simulink model "lab_hall"  (R2024b)
settings: Solver=FixedStepAuto  StartTime=0.0  StopTime=inf  FixedStep=0.001  RelTol=1e-3  EnableMultiTasking=on
libraries: stm32f4xxblockslib x2, simulink x1
settings Model: STM32="{\"AnalogInput\":[{\"ID\":\"lab_1:1\"},{\"ID\":\"lab_hall:1\"}],\"DigitalPortRead\":[{\"ID\":\"lab_1:126\"},{\"ID\":\"lab_hall:126\"}]}"  Creator=A1nz_01  LastModifiedBy=A1nz_01
settings OptimizationCC: EnhancedBackFolding=on  PassReuseOutputArgsAs=Individual arguments  ZeroExternalMemoryAtStartup=off  ZeroInternalMemoryAtStartup=off  MaxStackSize=64  OptimizeBlockOrder=speed  DifferentSizesBufferReuse=on  OptimizationCustomize=off  EfficientTunableParamExpr=on
settings DebuggingCC: ParameterTunabilityLossMsg=error
settings HardwareCC: ProdBitPerPointer=32  ProdBitPerSizeT=32  ProdBitPerPtrDiffT=32  ProdLargestAtomicInteger=Long  ProdLargestAtomicFloat=Double  ProdWordSize=32  ProdLongLongMode=on  ProdHWDeviceType=ARM Compatible->ARM Cortex-M
settings SFSimCC: MATLABDynamicMemAlloc=off
settings RTWCC: Description=Embedded Coder  SystemTargetFile=ert.tlc  HardwareBoard=STM32G4xx Based  TemplateMakefile=ert_default_tmf  Toolchain=GNU Tools for ARM Embedded Processors
settings CodeAppCC: ForceParamTrailComments=on  IgnoreCustomStorageClasses=off  OperatorAnnotations=on  SimulinkDataObjDesc=on  SFDataObjDesc=on  InsertBlockDesc=on
settings ERTTargetCC: TargetLangStandard=C99 (ISO)  CodeReplacementLibrary=ARM Cortex-M  ExtModeTransport=3  ExtModeStaticAlloc=on  ExtModeStaticAllocSize=2048  ExtModeMexFile=ext_xcp  ExtModeIntrfLevel=Level2 - Open  InlinedParameterPlacement=Hierarchical  DynamicArrayContainerType=coder::array

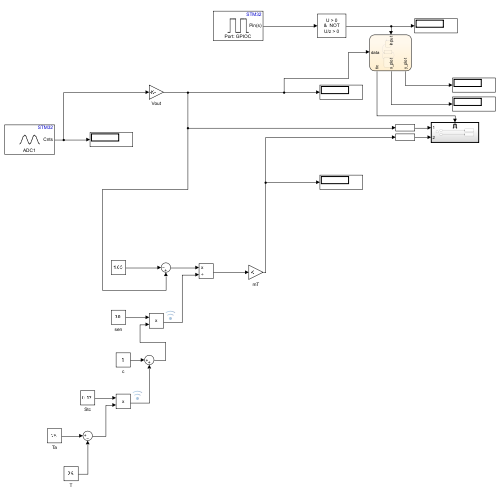
[thumbnail: Simulink's stored preview of the top-level diagram]
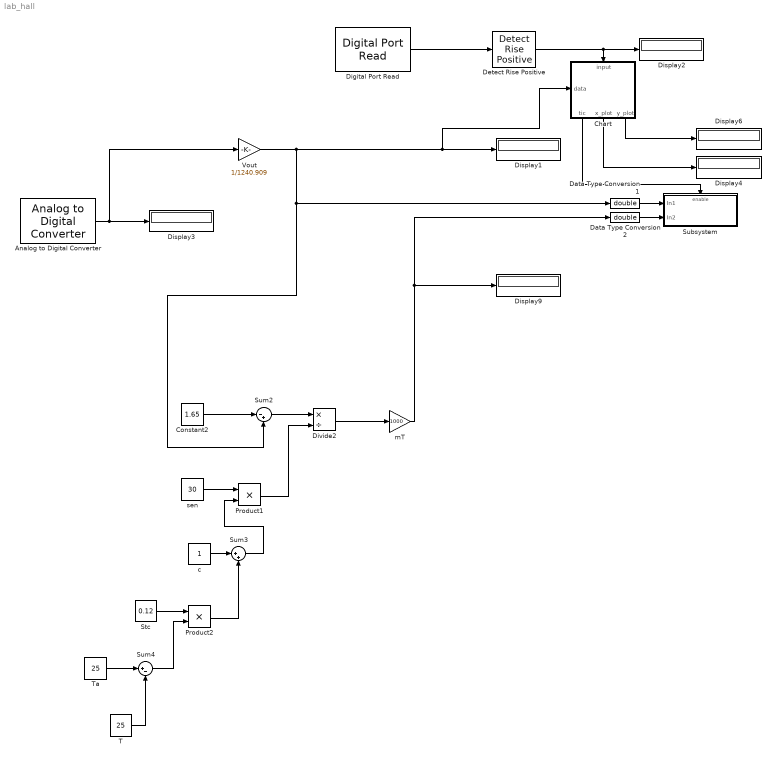
== system lab_hall ==
  Analog to Digital Converter : stm32f4xxblockslib/Analog to Digital Converter  ADCModule=ADC1  ConversionGroup=Regular  TriggerMode=Trigger and read  NumberOfConversions=1  EnableBufferConv=off  BufferLength=1  OutputStatus=off  SampleTime=-1  EnableSimPort=off  hoistedMaskSrc=ECSoC/ECSimCodegen/Analog to Digital Converter
  Chart : Stateflow chart  TreatAsAtomicUnit=on
      settings: PortSchema="{\"entries\":[{\"content\":{\"sides\":[{\"content\":{\"connectorIds\":[\"In1\"]},\"type\":\"ConnectorPlacement.EquallySpacedRectSide\",\"uuid\":\"15421bba-938f-45a9-ad39-0fb1dc31f746\"},{\"content\":{\"side\":\"RIGHT\"},\"type\":\"ConnectorPlacement.EquallySpacedRectSide\",\"uuid\":\"6df644a9-cb47-4d86-919b-b55e97b0d3b9\"},{\"content\":{\"connectorIds\":[\"In2\"],\"side\":\"TOP\"},\"type\":\"ConnectorPlacement.EquallySpacedRectSide\",\"uuid\":\"9fcc37fd-4916-48d6-817c-74b5556d6fa8\"},{\"content\":{\"connectorIds\":[\"Out1\",\"Out2\",\"Out3\"],\"side\":\"BOTTOM\"},\"type\":\"ConnectorPlacement.EquallySpacedRectSide\",\"uuid\":\"cb540dc6-d65e-4d03-87d2-789e1aed4831\"}]},\"type\":\"ConnectorPlacement.EquallySpacedConnector\",\"uuid\":\"c07b23df-6d95-4e9d-8fab-891c31dfc579\"}],\"packageUris\":[\"http://schema.mathworks.com/mf0/Connector/R2020b\"],\"version\":\"1.0\"}"
  Constant2 : Constant  Value=1.65
  Data Type Conversion1 : DataTypeConversion  OutDataTypeStr=double  SaturateOnIntegerOverflow=off  RndMeth=Floor
  Data Type Conversion2 : DataTypeConversion  OutDataTypeStr=double  SaturateOnIntegerOverflow=off  RndMeth=Floor
  Detect Rise Positive : simulink/Logic and Bit Operations/Detect Rise Positive  vinit=0  OutDataTypeStr=boolean
  Digital Port Read : stm32f4xxblockslib/Digital Port Read  PortName=GPIOC  PinNumber=[13]  ReadOperation=on  IOAsArray=on  SampleTime=-1  EnableSimPort=off  hoistedMaskSrc=ECSoC/ECSimCodegen/Digital Port Read
      settings: LibrarySourceBlock=stm32g4xxblockslib/Digital Port Read
  Display{1..4,6,9} (6 alike) : Display
  Divide2 : Product  Inputs=*/
  Product1 : Product
  Product2 : Product
  Stc : Constant  Value=0.12
  Subsystem : Subsystem
  Sum2 : Sum  Inputs=|-+
  Sum3 : Sum  Inputs=|++
  Sum4 : Sum  Inputs=|+-
  T : Constant  Value=25
  Ta : Constant  Value=25
  Vout : Gain  Gain=1/1240.909
  c : Constant
  mT : Gain  Gain=1000
  sen : Constant  Value=30
  wires:
  Analog to Digital Converter/1 -> Vout/1, Display3/1
  Vout/1 -> Chart/1(data), Display1/1, Data Type Conversion1/1, Sum2/2
  Digital Port Read/1 -> Detect Rise Positive/1
  Detect Rise Positive/1 -> Display2/1, Chart/2(input)
  Data Type Conversion1/1 -> Subsystem/1(In1)
  Data Type Conversion2/1 -> Subsystem/2(In2)
  Chart/1(tic) -> Subsystem/Enable
  Chart/2(x_plot) -> Display4/1
  Chart/3(y_plot) -> Display6/1
  Constant2/1 -> Sum2/1
  Sum2/1 -> Divide2/1
  sen/1 -> Product1/1
  c/1 -> Sum3/1
  Sum3/1 -> Product1/2
  Product2/1 -> Sum3/2
  Stc/1 -> Product2/1
  T/1 -> Sum4/2
  Sum4/1 -> Product2/2
  Ta/1 -> Sum4/1
  Product1/1 -> Divide2/2
  Divide2/1 -> mT/1
  mT/1 -> Display9/1, Data Type Conversion2/1

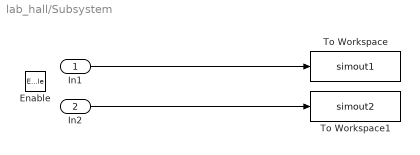
== system lab_hall/Subsystem ==
  In1 : Inport
  In2 : Inport  Port=2
  Enable : EnablePort
  To Workspace : ToWorkspace  VariableName=simout1  SampleTime=-1
      settings: Save2DSignal=2-D array (concatenate along first dimension)
  To Workspace1 : ToWorkspace  VariableName=simout2  SampleTime=-1
      settings: Save2DSignal=2-D array (concatenate along first dimension)
  wires:
  In1/1 -> To Workspace/1
  In2/1 -> To Workspace1/1

== stateflow chart lab_hall/Chart ==
  state setup
    loop = 0;
    tic = 0;
    x_plot = 0;
    y_plot = 0;
  state set
    loop = 0;
  state loop1
    entry:
    tic = 1;
    during:
    loop = loop + 0.001;
    exit:
    tic = 0;
    x_plot = x_plot + 2.77778
    y_plot = data
  (default) -> setup
  setup -> set
  loop1 -> set : [loop > 0.5 - 0.001]
  set -> loop1 : [input == 1]
  data: data input; input input; tic output; loop local; x_plot output; y_plot output
